simulink model "ModelRef"  (Simulink 9.1)
settings: Solver=FixedStepDiscrete  StartTime=0.0  StopTime=10.0  FixedStep=0.01  RelTol=1e-3
libraries: IOBlock_Library_TTC580 x2
settings Model: Creator=hokka  LastModifiedBy=hokka
settings DataIOCC: LimitDataPoints=on  SignalLoggingSaveFormat=ModelDataLogs
settings OptimizationCC: DefaultParameterBehavior=Inlined  ExpressionDepthLimit=2147483647  InitFltsAndDblsToZero=on  LifeSpan=1
settings DebuggingCC: SolverPrmCheckMsg=warning  InheritedTsInSrcMsg=none  FcnCallInpInsideContextMsg=warning  StateNameClashWarn=warning
settings HardwareCC: ProdLargestAtomicInteger=Long  ProdLargestAtomicFloat=Double  ProdIntDivRoundTo=Zero  ProdEndianess=BigEndian  ProdHWDeviceType=Texas Instruments->TMS570 Cortex-R4  TargetIntDivRoundTo=Zero  TargetEndianess=BigEndian  TargetHWDeviceType=Generic->32-bit Embedded Processor
settings SFSimCC: MATLABDynamicMemAlloc=off
settings RTWCC: SystemTargetFile=ert.tlc  GenCodeOnly=on  TemplateMakefile=ert_TTC580.tmf  Description=Real-Time Workshop Embedded Coder (no auto configuration)
settings CodeAppCC: IgnoreCustomStorageClasses=off  CustomSymbolStrType=$N$R$M  InternalIdentifier=Classic
settings ERTTargetCC: MultiwordLength=2048  SupportAbsoluteTime=off  SupportNonFinite=off  InlinedParameterPlacement=NonHierarchical  ERTCustomFileTemplate=example_file_process.tlc  ConvertIfToSwitch=off  SuppressUnreachableDefaultCases=off
settings ConfigComp: CovSFcnEnable=off

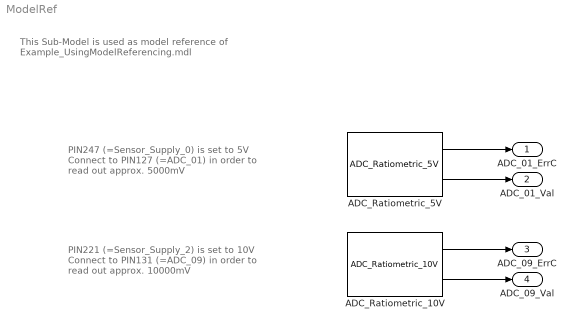
== system ModelRef ==
  note: PIN247 (=Sensor_Supply_0) is set to 5V
      | Connect to PIN127 (=ADC_01) in order to
      | read out approx. 5000mV
  note: PIN221 (=Sensor_Supply_2) is set to 10V
      | Connect to PIN131 (=ADC_09) in order to
      | read out approx. 10000mV
  note: This Sub-Model is used
      | as model reference of
      | Example_UsingModelReferencing.mdl
  ADC_Ratiometric_10V : IOBlock_Library_TTC580/ADC Blocks TTC580 IOlib/ADC_Ratiometric_10V  SampleTime=-1  ttlib=IO_Blk_Lib_TTC500  ttDescription=ADC_Ratiometric_10V  tt_iolib_version=0.17  adc_channel=IO_ADC_09  adc_type=IO_ADC_RATIOMETRIC  range=IO_ADC_RANGE_10V  pupd=IO_ADC_NO_PULL  sensor_supply=IO_SENSOR_SUPPLY_2  volt_sensor_supply=IO_POWER_ON_10V
      settings: SourceProductName=I/O Blocklibrary for TTC580
  ADC_Ratiometric_5V : IOBlock_Library_TTC580/ADC Blocks TTC580 IOlib/ADC_Ratiometric_5V  SampleTime=-1  ttlib=IO_Blk_Lib_TTC500  ttDescription=ADC_Ratiometric_5V  tt_iolib_version=0.17  adc_channel=IO_ADC_01  adc_type=IO_ADC_RATIOMETRIC  range=IO_ADC_RANGE_5V  pupd=IO_ADC_NO_PULL  sensor_supply=IO_SENSOR_SUPPLY_0
      settings: SourceProductName=I/O Blocklibrary for TTC580
  ADC_01_ErrC : Outport
  ADC_01_Val : Outport  Port=2
  ADC_09_ErrC : Outport  Port=3
  ADC_09_Val : Outport  Port=4
  wires:
  ADC_Ratiometric_5V/1 -> ADC_01_ErrC/1
  ADC_Ratiometric_5V/2 -> ADC_01_Val/1
  ADC_Ratiometric_10V/2 -> ADC_09_Val/1
  ADC_Ratiometric_10V/1 -> ADC_09_ErrC/1
